simulink library "halout"  (R2021b)
settings: Solver=VariableStepAuto  StartTime=0.0  StopTime=10.0  RelTol=1e-3
undefined symbols (not defined in the file): C_TASK_5MS_S, FALSE, KHAL_CAN1FD1APS3E2E_flg, KHAL_CAN1FD1APS3TxReq_flg, KHAL_CAN1FD1VCU2E2E_flg, KHAL_CAN1FD1VCU2TxReq_flg, KHAL_CAN1FD1VCU3E2E_flg, KHAL_CAN1FD1VCU3TxReq_flg, KHAL_CAN1TxReq_flg, KHAL_CAN1VMCFCM1E2E_flg, KHAL_CAN1VMCFCM1TxReq_flg, KHAL_CAN2TxReq_flg, KHAL_CAN3FD3VCU1toNIDECTxReq_flg, KHAL_CAN3FD3VCU1TxReq_flg, KHAL_CAN3FD3VCU2E2E_flg, KHAL_CAN3FD3VCU2toNIDECE2E_flg, KHAL_CAN3FD3VCU2toNIDECTxReq_flg, KHAL_CAN3FD3VCU2TxReq_flg, KHAL_CAN3TxReq_flg, KHAL_CAN4FD4CE1000E2E_flg, KHAL_CAN4FD4CE1000TxReq_flg, KHAL_CAN4TxReq_flg, KHAL_CAN5TxReq_flg, KHAL_CAN6FD6APS3E2E_flg, KHAL_CAN6FD6APS3TxReq_flg, KHAL_CAN6FD6VCU2E2E_flg, KHAL_CAN6FD6VCU2TxReq_flg, KHAL_CAN6TxReq_flg, ONE_INT, TRUE, ZERO_INT
libraries: FVT_lib x551, simulink x244
(part 15 of 26)

== system halout/HAL_OUT/CAN1/FD1_THCM1_0x182/RrCoolantflow ==
  RrCoolantflow : Inport
  Data Type Conversion : DataTypeConversion  OutDataTypeStr=uint8  RndMeth=Round
  convert_out : FVT_lib/hal/convert_out  gain=0.25  offset=0
  CAN1_Rr_Coolantflow : Outport
  wires:
  Data Type Conversion/1 -> CAN1_Rr_Coolantflow/1
  convert_out/1 -> Data Type Conversion/1
  RrCoolantflow/1 -> convert_out/1

== system halout/HAL_OUT/CAN1/FD1_THCM1_0x182/RrCoolanttemp ==
  RrCoolanttemp : Inport
  Data Type Conversion : DataTypeConversion  OutDataTypeStr=uint16  RndMeth=Round
  convert_out : FVT_lib/hal/convert_out  gain=1  offset=-40
  CAN1_Rr_Coolanttemp : Outport
  wires:
  Data Type Conversion/1 -> CAN1_Rr_Coolanttemp/1
  convert_out/1 -> Data Type Conversion/1
  RrCoolanttemp/1 -> convert_out/1

== system halout/HAL_OUT/CAN1/FD1_THCM1_0x182/sigAirIntenZon1St ==
  sigAirIntenZon1St : Inport
  Data Type Conversion : DataTypeConversion  OutDataTypeStr=uint8  RndMeth=Round
  CAN1_sigAirIntenZon1St : Outport
  wires:
  Data Type Conversion/1 -> CAN1_sigAirIntenZon1St/1
  sigAirIntenZon1St/1 -> Data Type Conversion/1

== system halout/HAL_OUT/CAN1/FD1_THCM1_0x182/sigAirIntenZon3St ==
  sigAirIntenZon3St : Inport
  Data Type Conversion : DataTypeConversion  OutDataTypeStr=uint8  RndMeth=Round
  CAN1_sigAirIntenZon3St : Outport
  wires:
  Data Type Conversion/1 -> CAN1_sigAirIntenZon3St/1
  sigAirIntenZon3St/1 -> Data Type Conversion/1

== system halout/HAL_OUT/CAN1/FD1_THCM1_0x182/sigAmbAirT ==
  sigAmbAirT : Inport
  Data Type Conversion : DataTypeConversion  OutDataTypeStr=uint8  RndMeth=Round
  convert_out : FVT_lib/hal/convert_out  gain=0.5  offset=-40
  CAN1_sigAmbAirT : Outport
  wires:
  Data Type Conversion/1 -> CAN1_sigAmbAirT/1
  convert_out/1 -> Data Type Conversion/1
  sigAmbAirT/1 -> convert_out/1

== system halout/HAL_OUT/CAN1/FD1_THCM1_0x182/sigCbnAirT ==
  sigCbnAirT : Inport
  Data Type Conversion : DataTypeConversion  OutDataTypeStr=uint8  RndMeth=Round
  convert_out : FVT_lib/hal/convert_out  gain=0.5  offset=-40
  CAN1_sigCbnAirT : Outport
  wires:
  Data Type Conversion/1 -> CAN1_sigCbnAirT/1
  convert_out/1 -> Data Type Conversion/1
  sigCbnAirT/1 -> convert_out/1

== system halout/HAL_OUT/CAN1/FD1_THCM1_0x182/sigCbnPTCPwrAct ==
  sigCbnPTCPwrAct : Inport
  Data Type Conversion : DataTypeConversion  OutDataTypeStr=uint8  RndMeth=Round
  convert_out : FVT_lib/hal/convert_out  gain=50  offset=0
  CAN1_sigCbnPTCPwrAct : Outport
  wires:
  Data Type Conversion/1 -> CAN1_sigCbnPTCPwrAct/1
  convert_out/1 -> Data Type Conversion/1
  sigCbnPTCPwrAct/1 -> convert_out/1

== system halout/HAL_OUT/CAN1/FD1_THCM1_0x182/sigCbnSolarLeft ==
  sigCbnSolarLeft : Inport
  Data Type Conversion : DataTypeConversion  OutDataTypeStr=uint8  RndMeth=Round
  convert_out : FVT_lib/hal/convert_out  gain=5  offset=0
  CAN1_sigCbnSolarLeft : Outport
  wires:
  Data Type Conversion/1 -> CAN1_sigCbnSolarLeft/1
  convert_out/1 -> Data Type Conversion/1
  sigCbnSolarLeft/1 -> convert_out/1

== system halout/HAL_OUT/CAN1/FD1_THCM1_0x182/sigCbnSolarRight ==
  sigCbnSolarRight : Inport
  Data Type Conversion : DataTypeConversion  OutDataTypeStr=uint8  RndMeth=Round
  convert_out : FVT_lib/hal/convert_out  gain=5  offset=0
  CAN1_sigCbnSolarRight : Outport
  wires:
  Data Type Conversion/1 -> CAN1_sigCbnSolarRight/1
  convert_out/1 -> Data Type Conversion/1
  sigCbnSolarRight/1 -> convert_out/1

== system halout/HAL_OUT/CAN1/FD1_THCM1_0x182/sigClmtCmprPwrAct ==
  sigClmtCmprPwrAct : Inport
  Data Type Conversion : DataTypeConversion  OutDataTypeStr=uint8  RndMeth=Round
  convert_out : FVT_lib/hal/convert_out  gain=50  offset=0
  CAN1_sigClmtCmprPwrAct : Outport
  wires:
  Data Type Conversion/1 -> CAN1_sigClmtCmprPwrAct/1
  convert_out/1 -> Data Type Conversion/1
  sigClmtCmprPwrAct/1 -> convert_out/1

== system halout/HAL_OUT/CAN1/FD1_THCM1_0x182/sigClntTHvBattOut ==
  sigClntTHvBattOut : Inport
  Data Type Conversion : DataTypeConversion  OutDataTypeStr=uint8  RndMeth=Round
  convert_out : FVT_lib/hal/convert_out  gain=0.5  offset=-40
  CAN1_sigClntTHvBattOut : Outport
  wires:
  Data Type Conversion/1 -> CAN1_sigClntTHvBattOut/1
  convert_out/1 -> Data Type Conversion/1
  sigClntTHvBattOut/1 -> convert_out/1

== system halout/HAL_OUT/CAN1/FD1_THCM1_0x182/sigDfrstSt ==
  sigDfrstSt : Inport
  Data Type Conversion : DataTypeConversion  OutDataTypeStr=uint8  RndMeth=Round
  CAN1_sigDfrstSt : Outport
  wires:
  Data Type Conversion/1 -> CAN1_sigDfrstSt/1
  sigDfrstSt/1 -> Data Type Conversion/1

== system halout/HAL_OUT/CAN1/FD1_THCM1_0x182/sigHvacSt ==
  sigHvacSt : Inport
  Data Type Conversion : DataTypeConversion  OutDataTypeStr=uint8  RndMeth=Round
  CAN1_sigHvacSt : Outport
  wires:
  Data Type Conversion/1 -> CAN1_sigHvacSt/1
  sigHvacSt/1 -> Data Type Conversion/1

== system halout/HAL_OUT/CAN1/FD1_THCM1_0x182/sigRecircSt ==
  sigRecircSt : Inport
  Data Type Conversion : DataTypeConversion  OutDataTypeStr=uint8  RndMeth=Round
  CAN1_sigRecircSt : Outport
  wires:
  Data Type Conversion/1 -> CAN1_sigRecircSt/1
  sigRecircSt/1 -> Data Type Conversion/1

== system halout/HAL_OUT/CAN1/FD1_THCM1_0x182/sigSetTempZon1St ==
  sigSetTempZon1St : Inport
  Data Type Conversion : DataTypeConversion  OutDataTypeStr=uint8  RndMeth=Round
  convert_out : FVT_lib/hal/convert_out  gain=0.5  offset=17
  CAN1_sigSetTempZon1St : Outport
  wires:
  Data Type Conversion/1 -> CAN1_sigSetTempZon1St/1
  convert_out/1 -> Data Type Conversion/1
  sigSetTempZon1St/1 -> convert_out/1

== system halout/HAL_OUT/CAN1/FD1_THCM1_0x182/sigSetTempZon2St ==
  sigSetTempZon2St : Inport
  Data Type Conversion : DataTypeConversion  OutDataTypeStr=uint8  RndMeth=Round
  convert_out : FVT_lib/hal/convert_out  gain=0.5  offset=17
  CAN1_sigSetTempZon2St : Outport
  wires:
  Data Type Conversion/1 -> CAN1_sigSetTempZon2St/1
  convert_out/1 -> Data Type Conversion/1
  sigSetTempZon2St/1 -> convert_out/1

== system halout/HAL_OUT/CAN1/FD1_THCM1_0x182/sigSetTempZon3St ==
  sigSetTempZon3St : Inport
  Data Type Conversion : DataTypeConversion  OutDataTypeStr=uint8  RndMeth=Round
  convert_out : FVT_lib/hal/convert_out  gain=0.5  offset=17
  CAN1_sigSetTempZon3St : Outport
  wires:
  Data Type Conversion/1 -> CAN1_sigSetTempZon3St/1
  convert_out/1 -> Data Type Conversion/1
  sigSetTempZon3St/1 -> convert_out/1

== system halout/HAL_OUT/CAN1/FD1_THCM1_0x182/sigWindDirZon1St ==
  sigWindDirZon1St : Inport
  Data Type Conversion : DataTypeConversion  OutDataTypeStr=uint8  RndMeth=Round
  CAN1_sigWindDirZon1St : Outport
  wires:
  Data Type Conversion/1 -> CAN1_sigWindDirZon1St/1
  sigWindDirZon1St/1 -> Data Type Conversion/1

== system halout/HAL_OUT/CAN1/FD1_THCM1_0x182/sigWindDirZon3St ==
  sigWindDirZon3St : Inport
  Data Type Conversion : DataTypeConversion  OutDataTypeStr=uint8  RndMeth=Round
  CAN1_sigWindDirZon3St : Outport
  wires:
  Data Type Conversion/1 -> CAN1_sigWindDirZon3St/1
  sigWindDirZon3St/1 -> Data Type Conversion/1

== system halout/HAL_OUT/CAN1/FD1_VCU1_0x116/CCCrlSta ==
  CCCrlSta : Inport
  Data Type Conversion : DataTypeConversion  OutDataTypeStr=uint8  RndMeth=Round
  CAN1_CC_Crl_Sta : Outport
  wires:
  Data Type Conversion/1 -> CAN1_CC_Crl_Sta/1
  CCCrlSta/1 -> Data Type Conversion/1

== system halout/HAL_OUT/CAN1/FD1_VCU1_0x116/EngAGSCloseSta ==
  EngAGSCloseSta : Inport
  Data Type Conversion : DataTypeConversion  OutDataTypeStr=uint8  RndMeth=Round
  CAN1_Eng_AGSCloseSta : Outport
  wires:
  Data Type Conversion/1 -> CAN1_Eng_AGSCloseSta/1
  EngAGSCloseSta/1 -> Data Type Conversion/1

== system halout/HAL_OUT/CAN1/FD1_VCU1_0x116/EngActvDmpDisabSta ==
  EngActvDmpDisabSta : Inport
  Data Type Conversion : DataTypeConversion  OutDataTypeStr=uint8  RndMeth=Round
  CAN1_Eng_ActvDmpDisabSta : Outport
  wires:
  Data Type Conversion/1 -> CAN1_Eng_ActvDmpDisabSta/1
  EngActvDmpDisabSta/1 -> Data Type Conversion/1

== system halout/HAL_OUT/CAN1/FD1_VCU1_0x116/EngCoastDwSta ==
  EngCoastDwSta : Inport
  Data Type Conversion : DataTypeConversion  OutDataTypeStr=uint8  RndMeth=Round
  CAN1_Eng_CoastDwSta : Outport
  wires:
  Data Type Conversion/1 -> CAN1_Eng_CoastDwSta/1
  EngCoastDwSta/1 -> Data Type Conversion/1

== system halout/HAL_OUT/CAN1/FD1_VCU1_0x116/EngPwrLockSta ==
  EngPwrLockSta : Inport
  Data Type Conversion : DataTypeConversion  OutDataTypeStr=uint8  RndMeth=Round
  CAN1_Eng_PwrLockSta : Outport
  wires:
  Data Type Conversion/1 -> CAN1_Eng_PwrLockSta/1
  EngPwrLockSta/1 -> Data Type Conversion/1

== system halout/HAL_OUT/CAN1/FD1_VCU1_0x116/HVPwrSta ==
  HVPwrSta : Inport
  Data Type Conversion : DataTypeConversion  OutDataTypeStr=uint8  RndMeth=Round
  CAN1_HVPwrSta : Outport
  wires:
  Data Type Conversion/1 -> CAN1_HVPwrSta/1
  HVPwrSta/1 -> Data Type Conversion/1

== system halout/HAL_OUT/CAN1/FD1_VCU1_0x116/LVPwrSta ==
  LVPwrSta : Inport
  Data Type Conversion : DataTypeConversion  OutDataTypeStr=uint8  RndMeth=Round
  CAN1_LVPwrSta : Outport
  wires:
  Data Type Conversion/1 -> CAN1_LVPwrSta/1
  LVPwrSta/1 -> Data Type Conversion/1

== system halout/HAL_OUT/CAN1/FD1_VCU1_0x116/MSACrlSta ==
  MSACrlSta : Inport
  Data Type Conversion : DataTypeConversion  OutDataTypeStr=uint8  RndMeth=Round
  CAN1_MSA_Crl_Sta : Outport
  wires:
  Data Type Conversion/1 -> CAN1_MSA_Crl_Sta/1
  MSACrlSta/1 -> Data Type Conversion/1

== system halout/HAL_OUT/CAN1/FD1_VCU1_0x116/PButtonSta ==
  PButtonSta : Inport
  Data Type Conversion : DataTypeConversion  OutDataTypeStr=uint8  RndMeth=Round
  CAN1_P_Button_Sta : Outport
  wires:
  Data Type Conversion/1 -> CAN1_P_Button_Sta/1
  PButtonSta/1 -> Data Type Conversion/1

== system halout/HAL_OUT/CAN1/FD1_VCU1_0x116/PrkReq ==
  PrkReq : Inport
  Data Type Conversion : DataTypeConversion  OutDataTypeStr=uint8  RndMeth=Round
  CAN1_PrkReq : Outport
  wires:
  Data Type Conversion/1 -> CAN1_PrkReq/1
  PrkReq/1 -> Data Type Conversion/1

== system halout/HAL_OUT/CAN1/FD1_VCU1_0x116/PrkReqValid ==
  PrkReqValid : Inport
  Data Type Conversion : DataTypeConversion  OutDataTypeStr=uint8  RndMeth=Round
  CAN1_PrkReqValid : Outport
  wires:
  Data Type Conversion/1 -> CAN1_PrkReqValid/1
  PrkReqValid/1 -> Data Type Conversion/1

== system halout/HAL_OUT/CAN1/FD1_VCU1_0x116/PwrSta ==
  PwrSta : Inport
  Data Type Conversion : DataTypeConversion  OutDataTypeStr=uint8  RndMeth=Round
  CAN1_PwrSta : Outport
  wires:
  Data Type Conversion/1 -> CAN1_PwrSta/1
  PwrSta/1 -> Data Type Conversion/1

== system halout/HAL_OUT/CAN1/FD1_VCU1_0x116/ShiftGearPosn ==
  ShiftGearPosn : Inport
  Data Type Conversion : DataTypeConversion  OutDataTypeStr=uint8  RndMeth=Round
  CAN1_ShiftGearPosn : Outport
  wires:
  Data Type Conversion/1 -> CAN1_ShiftGearPosn/1
  ShiftGearPosn/1 -> Data Type Conversion/1

== system halout/HAL_OUT/CAN1/FD1_VCU1_0x116/VehMalfunLevel ==
  VehMalfunLevel : Inport
  Data Type Conversion : DataTypeConversion  OutDataTypeStr=uint8  RndMeth=Round
  CAN1_VehMalfunLevel : Outport
  wires:
  Data Type Conversion/1 -> CAN1_VehMalfunLevel/1
  VehMalfunLevel/1 -> Data Type Conversion/1

== system halout/HAL_OUT/CAN1/FD1_VCU1_0x116/XWDMode ==
  XWDMode : Inport
  Data Type Conversion : DataTypeConversion  OutDataTypeStr=uint8  RndMeth=Round
  CAN1_XWDMode : Outport
  wires:
  Data Type Conversion/1 -> CAN1_XWDMode/1
  XWDMode/1 -> Data Type Conversion/1

== system halout/HAL_OUT/CAN1/FD1_VCU2_0x154/ACCCtrlAvail ==
  ACCCtrlAvail : Inport
  Data Type Conversion : DataTypeConversion  OutDataTypeStr=uint8  RndMeth=Round
  CAN1_ACC_CtrlAvail : Outport
  wires:
  Data Type Conversion/1 -> CAN1_ACC_CtrlAvail/1
  ACCCtrlAvail/1 -> Data Type Conversion/1

== system halout/HAL_OUT/CAN1/FD1_VCU2_0x154/AccPedalOverride ==
  AccPedalOverride : Inport
  Data Type Conversion : DataTypeConversion  OutDataTypeStr=uint8  RndMeth=Round
  CAN1_AccPedal_Override : Outport
  wires:
  Data Type Conversion/1 -> CAN1_AccPedal_Override/1
  AccPedalOverride/1 -> Data Type Conversion/1

== system halout/HAL_OUT/CAN1/FD1_VCU2_0x154/ActAPSPosn ==
  ActAPSPosn : Inport
  Data Type Conversion : DataTypeConversion  OutDataTypeStr=uint8  RndMeth=Round
  convert_out : FVT_lib/hal/convert_out  gain=0.394  offset=0
  CAN1_ActAPSPosn : Outport
  wires:
  Data Type Conversion/1 -> CAN1_ActAPSPosn/1
  convert_out/1 -> Data Type Conversion/1
  ActAPSPosn/1 -> convert_out/1

== system halout/HAL_OUT/CAN1/FD1_VCU2_0x154/Byte_0 ==
  CS_VCU2_CAN1 : Inport
  BitwiseOR : simulink/Logic and Bit Operations/Bitwise Operator  logicop=OR  UseBitMask=off  BitMask=bin2dec('11011001')  BitMaskRealWorld=Stored Integer
  SignalPack : FVT_lib/hal/SignalPack  RightShiftCnt=0  BitMask=2^8-1  LeftShiftCnt=0
  UnitConverter : DataTypeConversion  OutDataTypeStr=uint8  RndMeth=Round
  UnitConverter1 : DataTypeConversion  OutDataTypeStr=uint8  RndMeth=Round
  Byte_0 : Outport
  wires:
  BitwiseOR/1 -> Byte_0/1
  UnitConverter/1 -> BitwiseOR/1
  SignalPack/1 -> UnitConverter/1
  UnitConverter1/1 -> SignalPack/1
  CS_VCU2_CAN1/1 -> UnitConverter1/1

== system halout/HAL_OUT/CAN1/FD1_VCU2_0x154/Byte_1 ==
  RC_VCU2_CAN1 : Inport
  BitwiseOR : simulink/Logic and Bit Operations/Bitwise Operator  logicop=OR  UseBitMask=off  BitMask=bin2dec('11011001')  BitMaskRealWorld=Stored Integer
  SignalPack : FVT_lib/hal/SignalPack  RightShiftCnt=0  BitMask=2^4-1  LeftShiftCnt=0
  UnitConverter : DataTypeConversion  OutDataTypeStr=uint8  RndMeth=Round
  UnitConverter1 : DataTypeConversion  OutDataTypeStr=uint8  RndMeth=Round
  Byte_1 : Outport
  wires:
  BitwiseOR/1 -> Byte_1/1
  UnitConverter/1 -> BitwiseOR/1
  SignalPack/1 -> UnitConverter/1
  UnitConverter1/1 -> SignalPack/1
  RC_VCU2_CAN1/1 -> UnitConverter1/1

== system halout/HAL_OUT/CAN1/FD1_VCU2_0x154/Byte_10 ==
  VehActPwr : Inport
  BitwiseOR : simulink/Logic and Bit Operations/Bitwise Operator  logicop=OR  UseBitMask=off  BitMask=bin2dec('11011001')  BitMaskRealWorld=Stored Integer
  SignalPack : FVT_lib/hal/SignalPack  RightShiftCnt=16  BitMask=2^8-1  LeftShiftCnt=0
  UnitConverter : DataTypeConversion  OutDataTypeStr=uint8  RndMeth=Round
  UnitConverter1 : DataTypeConversion  OutDataTypeStr=uint32  RndMeth=Round
  convert_out : FVT_lib/hal/convert_out  gain=1  offset=-600000
  Byte_10 : Outport
  wires:
  BitwiseOR/1 -> Byte_10/1
  UnitConverter/1 -> BitwiseOR/1
  SignalPack/1 -> UnitConverter/1
  UnitConverter1/1 -> SignalPack/1
  convert_out/1 -> UnitConverter1/1
  VehActPwr/1 -> convert_out/1

== system halout/HAL_OUT/CAN1/FD1_VCU2_0x154/Byte_11 ==
  VehActPwr : Inport
  BitwiseOR : simulink/Logic and Bit Operations/Bitwise Operator  logicop=OR  UseBitMask=off  BitMask=bin2dec('11011001')  BitMaskRealWorld=Stored Integer
  SignalPack : FVT_lib/hal/SignalPack  RightShiftCnt=8  BitMask=2^8-1  LeftShiftCnt=0
  UnitConverter : DataTypeConversion  OutDataTypeStr=uint8  RndMeth=Round
  UnitConverter1 : DataTypeConversion  OutDataTypeStr=uint32  RndMeth=Round
  convert_out : FVT_lib/hal/convert_out  gain=1  offset=-600000
  Byte_11 : Outport
  wires:
  BitwiseOR/1 -> Byte_11/1
  UnitConverter/1 -> BitwiseOR/1
  SignalPack/1 -> UnitConverter/1
  UnitConverter1/1 -> SignalPack/1
  convert_out/1 -> UnitConverter1/1
  VehActPwr/1 -> convert_out/1

== system halout/HAL_OUT/CAN1/FD1_VCU2_0x154/Byte_12 ==
  VehActPwr : Inport
  BitwiseOR : simulink/Logic and Bit Operations/Bitwise Operator  logicop=OR  UseBitMask=off  BitMask=bin2dec('11011001')  BitMaskRealWorld=Stored Integer
  SignalPack : FVT_lib/hal/SignalPack  RightShiftCnt=0  BitMask=2^8-1  LeftShiftCnt=0
  UnitConverter : DataTypeConversion  OutDataTypeStr=uint8  RndMeth=Round
  UnitConverter1 : DataTypeConversion  OutDataTypeStr=uint32  RndMeth=Round
  convert_out : FVT_lib/hal/convert_out  gain=1  offset=-600000
  Byte_12 : Outport
  wires:
  BitwiseOR/1 -> Byte_12/1
  UnitConverter/1 -> BitwiseOR/1
  SignalPack/1 -> UnitConverter/1
  UnitConverter1/1 -> SignalPack/1
  convert_out/1 -> UnitConverter1/1
  VehActPwr/1 -> convert_out/1

== system halout/HAL_OUT/CAN1/FD1_VCU2_0x154/Byte_13 ==
  DriverTq : Inport
  BitwiseOR : simulink/Logic and Bit Operations/Bitwise Operator  logicop=OR  UseBitMask=off  BitMask=bin2dec('11011001')  BitMaskRealWorld=Stored Integer
  SignalPack : FVT_lib/hal/SignalPack  RightShiftCnt=8  BitMask=2^8-1  LeftShiftCnt=0
  UnitConverter : DataTypeConversion  OutDataTypeStr=uint8  RndMeth=Round
  UnitConverter1 : DataTypeConversion  OutDataTypeStr=uint16  RndMeth=Round
  convert_out : FVT_lib/hal/convert_out  gain=1  offset=-4300
  Byte_13 : Outport
  wires:
  BitwiseOR/1 -> Byte_13/1
  UnitConverter/1 -> BitwiseOR/1
  SignalPack/1 -> UnitConverter/1
  UnitConverter1/1 -> SignalPack/1
  convert_out/1 -> UnitConverter1/1
  DriverTq/1 -> convert_out/1

== system halout/HAL_OUT/CAN1/FD1_VCU2_0x154/Byte_14 ==
  DriverTq : Inport
  BitwiseOR : simulink/Logic and Bit Operations/Bitwise Operator  logicop=OR  UseBitMask=off  BitMask=bin2dec('11011001')  BitMaskRealWorld=Stored Integer
  SignalPack : FVT_lib/hal/SignalPack  RightShiftCnt=0  BitMask=2^8-1  LeftShiftCnt=0
  UnitConverter : DataTypeConversion  OutDataTypeStr=uint8  RndMeth=Round
  UnitConverter1 : DataTypeConversion  OutDataTypeStr=uint16  RndMeth=Round
  convert_out : FVT_lib/hal/convert_out  gain=1  offset=-4300
  Byte_14 : Outport
  wires:
  BitwiseOR/1 -> Byte_14/1
  UnitConverter/1 -> BitwiseOR/1
  SignalPack/1 -> UnitConverter/1
  UnitConverter1/1 -> SignalPack/1
  convert_out/1 -> UnitConverter1/1
  DriverTq/1 -> convert_out/1

== system halout/HAL_OUT/CAN1/FD1_VCU2_0x154/Byte_15 ==
  ActAPSPosn : Inport
  BitwiseOR : simulink/Logic and Bit Operations/Bitwise Operator  logicop=OR  UseBitMask=off  BitMask=bin2dec('11011001')  BitMaskRealWorld=Stored Integer
  SignalPack : FVT_lib/hal/SignalPack  RightShiftCnt=0  BitMask=2^8-1  LeftShiftCnt=0
  UnitConverter : DataTypeConversion  OutDataTypeStr=uint8  RndMeth=Round
  UnitConverter1 : DataTypeConversion  OutDataTypeStr=uint8  RndMeth=Round
  convert_out : FVT_lib/hal/convert_out  gain=0.394  offset=0
  Byte_15 : Outport
  wires:
  BitwiseOR/1 -> Byte_15/1
  UnitConverter/1 -> BitwiseOR/1
  SignalPack/1 -> UnitConverter/1
  UnitConverter1/1 -> SignalPack/1
  convert_out/1 -> UnitConverter1/1
  ActAPSPosn/1 -> convert_out/1

== system halout/HAL_OUT/CAN1/FD1_VCU2_0x154/Byte_2 ==
  Fr_DriverTq : Inport
  BitwiseOR : simulink/Logic and Bit Operations/Bitwise Operator  logicop=OR  UseBitMask=off  BitMask=bin2dec('11011001')  BitMaskRealWorld=Stored Integer
  SignalPack : FVT_lib/hal/SignalPack  RightShiftCnt=8  BitMask=2^8-1  LeftShiftCnt=0
  UnitConverter : DataTypeConversion  OutDataTypeStr=uint8  RndMeth=Round
  UnitConverter1 : DataTypeConversion  OutDataTypeStr=uint16  RndMeth=Round
  convert_out : FVT_lib/hal/convert_out  gain=0.5  offset=-5300
  Byte_2 : Outport
  wires:
  BitwiseOR/1 -> Byte_2/1
  UnitConverter/1 -> BitwiseOR/1
  SignalPack/1 -> UnitConverter/1
  UnitConverter1/1 -> SignalPack/1
  convert_out/1 -> UnitConverter1/1
  Fr_DriverTq/1 -> convert_out/1

== system halout/HAL_OUT/CAN1/FD1_VCU2_0x154/Byte_3 ==
  Fr_DriverTq : Inport
  BitwiseOR : simulink/Logic and Bit Operations/Bitwise Operator  logicop=OR  UseBitMask=off  BitMask=bin2dec('11011001')  BitMaskRealWorld=Stored Integer
  SignalPack : FVT_lib/hal/SignalPack  RightShiftCnt=0  BitMask=2^8-1  LeftShiftCnt=0
  UnitConverter : DataTypeConversion  OutDataTypeStr=uint8  RndMeth=Round
  UnitConverter1 : DataTypeConversion  OutDataTypeStr=uint16  RndMeth=Round
  convert_out : FVT_lib/hal/convert_out  gain=0.5  offset=-5300
  Byte_3 : Outport
  wires:
  BitwiseOR/1 -> Byte_3/1
  UnitConverter/1 -> BitwiseOR/1
  SignalPack/1 -> UnitConverter/1
  UnitConverter1/1 -> SignalPack/1
  convert_out/1 -> UnitConverter1/1
  Fr_DriverTq/1 -> convert_out/1

== system halout/HAL_OUT/CAN1/FD1_VCU2_0x154/Byte_4 ==
  Rr_DriverTq : Inport
  BitwiseOR : simulink/Logic and Bit Operations/Bitwise Operator  logicop=OR  UseBitMask=off  BitMask=bin2dec('11011001')  BitMaskRealWorld=Stored Integer
  SignalPack : FVT_lib/hal/SignalPack  RightShiftCnt=8  BitMask=2^8-1  LeftShiftCnt=0
  UnitConverter : DataTypeConversion  OutDataTypeStr=uint8  RndMeth=Round
  UnitConverter1 : DataTypeConversion  OutDataTypeStr=uint16  RndMeth=Round
  convert_out : FVT_lib/hal/convert_out  gain=0.5  offset=-5300
  Byte_4 : Outport
  wires:
  BitwiseOR/1 -> Byte_4/1
  UnitConverter/1 -> BitwiseOR/1
  SignalPack/1 -> UnitConverter/1
  UnitConverter1/1 -> SignalPack/1
  convert_out/1 -> UnitConverter1/1
  Rr_DriverTq/1 -> convert_out/1

== system halout/HAL_OUT/CAN1/FD1_VCU2_0x154/Byte_5 ==
  Rr_DriverTq : Inport
  BitwiseOR : simulink/Logic and Bit Operations/Bitwise Operator  logicop=OR  UseBitMask=off  BitMask=bin2dec('11011001')  BitMaskRealWorld=Stored Integer
  SignalPack : FVT_lib/hal/SignalPack  RightShiftCnt=0  BitMask=2^8-1  LeftShiftCnt=0
  UnitConverter : DataTypeConversion  OutDataTypeStr=uint8  RndMeth=Round
  UnitConverter1 : DataTypeConversion  OutDataTypeStr=uint16  RndMeth=Round
  convert_out : FVT_lib/hal/convert_out  gain=0.5  offset=-5300
  Byte_5 : Outport
  wires:
  BitwiseOR/1 -> Byte_5/1
  UnitConverter/1 -> BitwiseOR/1
  SignalPack/1 -> UnitConverter/1
  UnitConverter1/1 -> SignalPack/1
  convert_out/1 -> UnitConverter1/1
  Rr_DriverTq/1 -> convert_out/1

== system halout/HAL_OUT/CAN1/FD1_VCU2_0x154/Byte_6 ==
  ACC_CtrlAvail : Inport
  AccPedal_Override : Inport  Port=2
  BitwiseOR : simulink/Logic and Bit Operations/Bitwise Operator  logicop=OR  UseBitMask=off  NumInputPorts=2  BitMask=bin2dec('11011001')  BitMaskRealWorld=Stored Integer
  SignalPack : FVT_lib/hal/SignalPack  RightShiftCnt=0  BitMask=2^1-1  LeftShiftCnt=7
  SignalPack1 : FVT_lib/hal/SignalPack  RightShiftCnt=0  BitMask=2^1-1  LeftShiftCnt=6
  UnitConverter{,1..3} (4 alike) : DataTypeConversion  OutDataTypeStr=uint8  RndMeth=Round
  Byte_6 : Outport
  wires:
  BitwiseOR/1 -> Byte_6/1
  UnitConverter/1 -> BitwiseOR/1
  SignalPack/1 -> UnitConverter/1
  UnitConverter1/1 -> SignalPack/1
  ACC_CtrlAvail/1 -> UnitConverter1/1
  UnitConverter2/1 -> BitwiseOR/2
  SignalPack1/1 -> UnitConverter2/1
  UnitConverter3/1 -> SignalPack1/1
  AccPedal_Override/1 -> UnitConverter3/1

== system halout/HAL_OUT/CAN1/FD1_VCU2_0x154/CRC8_IfAction_Tx ==
  CAN_E2E_flg : Inport
  DataID1 : Inport  Port=2
  DataID2 : Inport  Port=3
  RawData : Inport  Port=4
  Data Type Conversion : DataTypeConversion  OutDataTypeStr=uint8
  If : If
  If Action Subsystem : Subsystem  TreatAsAtomicUnit=on
  If Action Subsystem1 : Subsystem  TreatAsAtomicUnit=on
  Merge : Merge
  CRC8 : Outport
  wires:
  If/2 -> If Action Subsystem/Action
  If/1 -> If Action Subsystem1/Action
  CAN_E2E_flg/1 -> [CAN_E2E_flg]
  DataID1/1 -> [DataID1]
  DataID2/1 -> [DataID2]
  RawData/1 -> [RawData]
  [CAN_E2E_flg] -> Data Type Conversion/1
  [DataID1] -> If Action Subsystem1/1(CAN_E2E_ID1)
  [DataID2] -> If Action Subsystem1/2(CAN_E2E_ID2)
  [RawData] -> If Action Subsystem1/3(Byte1)
  [RawData] -> If Action Subsystem/1(Byte1)
  If Action Subsystem1/1(CRC8_E2EResult) -> Merge/1
  If Action Subsystem/1(CRC8_Result) -> Merge/2
  Merge/1 -> CRC8/1
  Data Type Conversion/1 -> If/1

== system halout/HAL_OUT/CAN1/FD1_VCU2_0x154/CSVCU2CAN1 ==
  CSVCU2CAN1 : Inport
  Data Type Conversion : DataTypeConversion  OutDataTypeStr=uint8  RndMeth=Round
  CAN1_CS_VCU2_CAN1 : Outport
  wires:
  Data Type Conversion/1 -> CAN1_CS_VCU2_CAN1/1
  CSVCU2CAN1/1 -> Data Type Conversion/1

== system halout/HAL_OUT/CAN1/FD1_VCU2_0x154/DriverTq ==
  DriverTq : Inport
  Data Type Conversion : DataTypeConversion  OutDataTypeStr=uint16  RndMeth=Round
  convert_out : FVT_lib/hal/convert_out  gain=1  offset=-4300
  CAN1_DriverTq : Outport
  wires:
  Data Type Conversion/1 -> CAN1_DriverTq/1
  convert_out/1 -> Data Type Conversion/1
  DriverTq/1 -> convert_out/1

== system halout/HAL_OUT/CAN1/FD1_VCU2_0x154/FrDriverTq ==
  FrDriverTq : Inport
  Data Type Conversion : DataTypeConversion  OutDataTypeStr=uint16  RndMeth=Round
  convert_out : FVT_lib/hal/convert_out  gain=0.5  offset=-5300
  CAN1_Fr_DriverTq : Outport
  wires:
  Data Type Conversion/1 -> CAN1_Fr_DriverTq/1
  convert_out/1 -> Data Type Conversion/1
  FrDriverTq/1 -> convert_out/1

== system halout/HAL_OUT/CAN1/FD1_VCU2_0x154/RCVCU2CAN1 ==
  RCVCU2CAN1 : Inport
  Data Type Conversion : DataTypeConversion  OutDataTypeStr=uint8  RndMeth=Round
  CAN1_RC_VCU2_CAN1 : Outport
  wires:
  Data Type Conversion/1 -> CAN1_RC_VCU2_CAN1/1
  RCVCU2CAN1/1 -> Data Type Conversion/1

== system halout/HAL_OUT/CAN1/FD1_VCU2_0x154/RrDriverTq ==
  RrDriverTq : Inport
  Data Type Conversion : DataTypeConversion  OutDataTypeStr=uint16  RndMeth=Round
  convert_out : FVT_lib/hal/convert_out  gain=0.5  offset=-5300
  CAN1_Rr_DriverTq : Outport
  wires:
  Data Type Conversion/1 -> CAN1_Rr_DriverTq/1
  convert_out/1 -> Data Type Conversion/1
  RrDriverTq/1 -> convert_out/1

== system halout/HAL_OUT/CAN1/FD1_VCU2_0x154/VehActPwr ==
  VehActPwr : Inport
  Data Type Conversion : DataTypeConversion  OutDataTypeStr=uint32  RndMeth=Round
  convert_out : FVT_lib/hal/convert_out  gain=1  offset=-600000
  CAN1_VehActPwr : Outport
  wires:
  Data Type Conversion/1 -> CAN1_VehActPwr/1
  convert_out/1 -> Data Type Conversion/1
  VehActPwr/1 -> convert_out/1

== system halout/HAL_OUT/CAN1/FD1_VCU3_0x159/Byte_0 ==
  CS_VCU3_CAN1 : Inport
  BitwiseOR : simulink/Logic and Bit Operations/Bitwise Operator  logicop=OR  UseBitMask=off  BitMask=bin2dec('11011001')  BitMaskRealWorld=Stored Integer
  SignalPack : FVT_lib/hal/SignalPack  RightShiftCnt=0  BitMask=2^8-1  LeftShiftCnt=0
  UnitConverter : DataTypeConversion  OutDataTypeStr=uint8  RndMeth=Round
  UnitConverter1 : DataTypeConversion  OutDataTypeStr=uint8  RndMeth=Round
  Byte_0 : Outport
  wires:
  BitwiseOR/1 -> Byte_0/1
  UnitConverter/1 -> BitwiseOR/1
  SignalPack/1 -> UnitConverter/1
  UnitConverter1/1 -> SignalPack/1
  CS_VCU3_CAN1/1 -> UnitConverter1/1

== system halout/HAL_OUT/CAN1/FD1_VCU3_0x159/Byte_1 ==
  RC_VCU3_CAN1 : Inport
  BitwiseOR : simulink/Logic and Bit Operations/Bitwise Operator  logicop=OR  UseBitMask=off  BitMask=bin2dec('11011001')  BitMaskRealWorld=Stored Integer
  SignalPack : FVT_lib/hal/SignalPack  RightShiftCnt=0  BitMask=2^4-1  LeftShiftCnt=0
  UnitConverter : DataTypeConversion  OutDataTypeStr=uint8  RndMeth=Round
  UnitConverter1 : DataTypeConversion  OutDataTypeStr=uint8  RndMeth=Round
  Byte_1 : Outport
  wires:
  BitwiseOR/1 -> Byte_1/1
  UnitConverter/1 -> BitwiseOR/1
  SignalPack/1 -> UnitConverter/1
  UnitConverter1/1 -> SignalPack/1
  RC_VCU3_CAN1/1 -> UnitConverter1/1

== system halout/HAL_OUT/CAN1/FD1_VCU3_0x159/Byte_10 ==
  Rr_EDURealDrvOrBRgnTq : Inport
  BitwiseOR : simulink/Logic and Bit Operations/Bitwise Operator  logicop=OR  UseBitMask=off  BitMask=bin2dec('11011001')  BitMaskRealWorld=Stored Integer
  SignalPack : FVT_lib/hal/SignalPack  RightShiftCnt=8  BitMask=2^8-1  LeftShiftCnt=0
  UnitConverter : DataTypeConversion  OutDataTypeStr=uint8  RndMeth=Round
  UnitConverter1 : DataTypeConversion  OutDataTypeStr=uint16  RndMeth=Round
  convert_out : FVT_lib/hal/convert_out  gain=0.5  offset=-5300
  Byte_10 : Outport
  wires:
  BitwiseOR/1 -> Byte_10/1
  UnitConverter/1 -> BitwiseOR/1
  SignalPack/1 -> UnitConverter/1
  UnitConverter1/1 -> SignalPack/1
  convert_out/1 -> UnitConverter1/1
  Rr_EDURealDrvOrBRgnTq/1 -> convert_out/1

== system halout/HAL_OUT/CAN1/FD1_VCU3_0x159/Byte_11 ==
  Rr_EDURealDrvOrBRgnTq : Inport
  BitwiseOR : simulink/Logic and Bit Operations/Bitwise Operator  logicop=OR  UseBitMask=off  BitMask=bin2dec('11011001')  BitMaskRealWorld=Stored Integer
  SignalPack : FVT_lib/hal/SignalPack  RightShiftCnt=0  BitMask=2^8-1  LeftShiftCnt=0
  UnitConverter : DataTypeConversion  OutDataTypeStr=uint8  RndMeth=Round
  UnitConverter1 : DataTypeConversion  OutDataTypeStr=uint16  RndMeth=Round
  convert_out : FVT_lib/hal/convert_out  gain=0.5  offset=-5300
  Byte_11 : Outport
  wires:
  BitwiseOR/1 -> Byte_11/1
  UnitConverter/1 -> BitwiseOR/1
  SignalPack/1 -> UnitConverter/1
  UnitConverter1/1 -> SignalPack/1
  convert_out/1 -> UnitConverter1/1
  Rr_EDURealDrvOrBRgnTq/1 -> convert_out/1

== system halout/HAL_OUT/CAN1/FD1_VCU3_0x159/Byte_12 ==
  Fr_EDUAvailBrkRgnTqValid : Inport
  Fr_EDUSpd : Inport  Port=2
  Rr_EDUAvailBrkRgnTqValid : Inport  Port=3
  BitwiseOR : simulink/Logic and Bit Operations/Bitwise Operator  logicop=OR  UseBitMask=off  NumInputPorts=3  BitMask=bin2dec('11011001')  BitMaskRealWorld=Stored Integer
  SignalPack : FVT_lib/hal/SignalPack  RightShiftCnt=0  BitMask=2^1-1  LeftShiftCnt=6
  SignalPack1 : FVT_lib/hal/SignalPack  RightShiftCnt=8  BitMask=2^4-1  LeftShiftCnt=0
  SignalPack2 : FVT_lib/hal/SignalPack  RightShiftCnt=0  BitMask=2^1-1  LeftShiftCnt=7
  UnitConverter{,1..2,4..5} (5 alike) : DataTypeConversion  OutDataTypeStr=uint8  RndMeth=Round
  UnitConverter3 : DataTypeConversion  OutDataTypeStr=uint16  RndMeth=Round
  convert_out : FVT_lib/hal/convert_out  gain=1  offset=-2000
  Byte_12 : Outport
  wires:
  BitwiseOR/1 -> Byte_12/1
  UnitConverter/1 -> BitwiseOR/1
  SignalPack/1 -> UnitConverter/1
  UnitConverter1/1 -> SignalPack/1
  Fr_EDUAvailBrkRgnTqValid/1 -> UnitConverter1/1
  UnitConverter2/1 -> BitwiseOR/2
  SignalPack1/1 -> UnitConverter2/1
  UnitConverter3/1 -> SignalPack1/1
  convert_out/1 -> UnitConverter3/1
  Fr_EDUSpd/1 -> convert_out/1
  UnitConverter4/1 -> BitwiseOR/3
  SignalPack2/1 -> UnitConverter4/1
  UnitConverter5/1 -> SignalPack2/1
  Rr_EDUAvailBrkRgnTqValid/1 -> UnitConverter5/1

== system halout/HAL_OUT/CAN1/FD1_VCU3_0x159/Byte_13 ==
  Fr_EDUSpd : Inport
  BitwiseOR : simulink/Logic and Bit Operations/Bitwise Operator  logicop=OR  UseBitMask=off  BitMask=bin2dec('11011001')  BitMaskRealWorld=Stored Integer
  SignalPack : FVT_lib/hal/SignalPack  RightShiftCnt=0  BitMask=2^8-1  LeftShiftCnt=0
  UnitConverter : DataTypeConversion  OutDataTypeStr=uint8  RndMeth=Round
  UnitConverter1 : DataTypeConversion  OutDataTypeStr=uint16  RndMeth=Round
  convert_out : FVT_lib/hal/convert_out  gain=1  offset=-2000
  Byte_13 : Outport
  wires:
  BitwiseOR/1 -> Byte_13/1
  UnitConverter/1 -> BitwiseOR/1
  SignalPack/1 -> UnitConverter/1
  UnitConverter1/1 -> SignalPack/1
  convert_out/1 -> UnitConverter1/1
  Fr_EDUSpd/1 -> convert_out/1

== system halout/HAL_OUT/CAN1/FD1_VCU3_0x159/Byte_14 ==
  Fr_EDURealARgnTq : Inport
  BitwiseOR : simulink/Logic and Bit Operations/Bitwise Operator  logicop=OR  UseBitMask=off  BitMask=bin2dec('11011001')  BitMaskRealWorld=Stored Integer
  SignalPack : FVT_lib/hal/SignalPack  RightShiftCnt=8  BitMask=2^8-1  LeftShiftCnt=0
  UnitConverter : DataTypeConversion  OutDataTypeStr=uint8  RndMeth=Round
  UnitConverter1 : DataTypeConversion  OutDataTypeStr=uint16  RndMeth=Round
  convert_out : FVT_lib/hal/convert_out  gain=1  offset=-5300
  Byte_14 : Outport
  wires:
  BitwiseOR/1 -> Byte_14/1
  UnitConverter/1 -> BitwiseOR/1
  SignalPack/1 -> UnitConverter/1
  UnitConverter1/1 -> SignalPack/1
  convert_out/1 -> UnitConverter1/1
  Fr_EDURealARgnTq/1 -> convert_out/1

== system halout/HAL_OUT/CAN1/FD1_VCU3_0x159/Byte_15 ==
  Fr_EDURealARgnTq : Inport
  BitwiseOR : simulink/Logic and Bit Operations/Bitwise Operator  logicop=OR  UseBitMask=off  BitMask=bin2dec('11011001')  BitMaskRealWorld=Stored Integer
  SignalPack : FVT_lib/hal/SignalPack  RightShiftCnt=0  BitMask=2^8-1  LeftShiftCnt=0
  UnitConverter : DataTypeConversion  OutDataTypeStr=uint8  RndMeth=Round
  UnitConverter1 : DataTypeConversion  OutDataTypeStr=uint16  RndMeth=Round
  convert_out : FVT_lib/hal/convert_out  gain=1  offset=-5300
  Byte_15 : Outport
  wires:
  BitwiseOR/1 -> Byte_15/1
  UnitConverter/1 -> BitwiseOR/1
  SignalPack/1 -> UnitConverter/1
  UnitConverter1/1 -> SignalPack/1
  convert_out/1 -> UnitConverter1/1
  Fr_EDURealARgnTq/1 -> convert_out/1

== system halout/HAL_OUT/CAN1/FD1_VCU3_0x159/Byte_16 ==
  Fr_EDUAvailBrkRgnTq : Inport
  BitwiseOR : simulink/Logic and Bit Operations/Bitwise Operator  logicop=OR  UseBitMask=off  BitMask=bin2dec('11011001')  BitMaskRealWorld=Stored Integer
  SignalPack : FVT_lib/hal/SignalPack  RightShiftCnt=8  BitMask=2^8-1  LeftShiftCnt=0
  UnitConverter : DataTypeConversion  OutDataTypeStr=uint8  RndMeth=Round
  UnitConverter1 : DataTypeConversion  OutDataTypeStr=uint16  RndMeth=Round
  convert_out : FVT_lib/hal/convert_out  gain=0.5  offset=-5300
  Byte_16 : Outport
  wires:
  BitwiseOR/1 -> Byte_16/1
  UnitConverter/1 -> BitwiseOR/1
  SignalPack/1 -> UnitConverter/1
  UnitConverter1/1 -> SignalPack/1
  convert_out/1 -> UnitConverter1/1
  Fr_EDUAvailBrkRgnTq/1 -> convert_out/1

== system halout/HAL_OUT/CAN1/FD1_VCU3_0x159/Byte_17 ==
  Fr_EDUAvailBrkRgnTq : Inport
  BitwiseOR : simulink/Logic and Bit Operations/Bitwise Operator  logicop=OR  UseBitMask=off  BitMask=bin2dec('11011001')  BitMaskRealWorld=Stored Integer
  SignalPack : FVT_lib/hal/SignalPack  RightShiftCnt=0  BitMask=2^8-1  LeftShiftCnt=0
  UnitConverter : DataTypeConversion  OutDataTypeStr=uint8  RndMeth=Round
  UnitConverter1 : DataTypeConversion  OutDataTypeStr=uint16  RndMeth=Round
  convert_out : FVT_lib/hal/convert_out  gain=0.5  offset=-5300
  Byte_17 : Outport
  wires:
  BitwiseOR/1 -> Byte_17/1
  UnitConverter/1 -> BitwiseOR/1
  SignalPack/1 -> UnitConverter/1
  UnitConverter1/1 -> SignalPack/1
  convert_out/1 -> UnitConverter1/1
  Fr_EDUAvailBrkRgnTq/1 -> convert_out/1

== system halout/HAL_OUT/CAN1/FD1_VCU3_0x159/Byte_18 ==
  Fr_EDURealDrvOrBRgnTq : Inport
  BitwiseOR : simulink/Logic and Bit Operations/Bitwise Operator  logicop=OR  UseBitMask=off  BitMask=bin2dec('11011001')  BitMaskRealWorld=Stored Integer
  SignalPack : FVT_lib/hal/SignalPack  RightShiftCnt=8  BitMask=2^8-1  LeftShiftCnt=0
  UnitConverter : DataTypeConversion  OutDataTypeStr=uint8  RndMeth=Round
  UnitConverter1 : DataTypeConversion  OutDataTypeStr=uint16  RndMeth=Round
  convert_out : FVT_lib/hal/convert_out  gain=0.5  offset=-5300
  Byte_18 : Outport
  wires:
  BitwiseOR/1 -> Byte_18/1
  UnitConverter/1 -> BitwiseOR/1
  SignalPack/1 -> UnitConverter/1
  UnitConverter1/1 -> SignalPack/1
  convert_out/1 -> UnitConverter1/1
  Fr_EDURealDrvOrBRgnTq/1 -> convert_out/1

== system halout/HAL_OUT/CAN1/FD1_VCU3_0x159/Byte_19 ==
  Fr_EDURealDrvOrBRgnTq : Inport
  BitwiseOR : simulink/Logic and Bit Operations/Bitwise Operator  logicop=OR  UseBitMask=off  BitMask=bin2dec('11011001')  BitMaskRealWorld=Stored Integer
  SignalPack : FVT_lib/hal/SignalPack  RightShiftCnt=0  BitMask=2^8-1  LeftShiftCnt=0
  UnitConverter : DataTypeConversion  OutDataTypeStr=uint8  RndMeth=Round
  UnitConverter1 : DataTypeConversion  OutDataTypeStr=uint16  RndMeth=Round
  convert_out : FVT_lib/hal/convert_out  gain=0.5  offset=-5300
  Byte_19 : Outport
  wires:
  BitwiseOR/1 -> Byte_19/1
  UnitConverter/1 -> BitwiseOR/1
  SignalPack/1 -> UnitConverter/1
  UnitConverter1/1 -> SignalPack/1
  convert_out/1 -> UnitConverter1/1
  Fr_EDURealDrvOrBRgnTq/1 -> convert_out/1

== system halout/HAL_OUT/CAN1/FD1_VCU3_0x159/Byte_3 ==
  Fr_EDUSpdValid : Inport
  Fr_RgnDecrSta : Inport  Port=2
  Fr_RgnPermSta : Inport  Port=3
  RgnAbnorSta : Inport  Port=4
  Rr_EDUSpdValid : Inport  Port=5
  Rr_RgnDecrSta : Inport  Port=6
  Rr_RgnPermSta : Inport  Port=7
  BitwiseOR : simulink/Logic and Bit Operations/Bitwise Operator  logicop=OR  UseBitMask=off  NumInputPorts=7  BitMask=bin2dec('11011001')  BitMaskRealWorld=Stored Integer
  SignalPack : FVT_lib/hal/SignalPack  RightShiftCnt=0  BitMask=2^1-1  LeftShiftCnt=6
  SignalPack1 : FVT_lib/hal/SignalPack  RightShiftCnt=0  BitMask=2^1-1  LeftShiftCnt=3
  SignalPack2 : FVT_lib/hal/SignalPack  RightShiftCnt=0  BitMask=2^1-1  LeftShiftCnt=1
  SignalPack3 : FVT_lib/hal/SignalPack  RightShiftCnt=0  BitMask=2^1-1  LeftShiftCnt=4
  SignalPack4 : FVT_lib/hal/SignalPack  RightShiftCnt=0  BitMask=2^1-1  LeftShiftCnt=5
  SignalPack5 : FVT_lib/hal/SignalPack  RightShiftCnt=0  BitMask=2^1-1  LeftShiftCnt=2
  SignalPack6 : FVT_lib/hal/SignalPack  RightShiftCnt=0  BitMask=2^1-1  LeftShiftCnt=0
  UnitConverter{,1..13} (14 alike) : DataTypeConversion  OutDataTypeStr=uint8  RndMeth=Round
  Byte_3 : Outport
  wires:
  BitwiseOR/1 -> Byte_3/1
  UnitConverter/1 -> BitwiseOR/1
  SignalPack/1 -> UnitConverter/1
  UnitConverter1/1 -> SignalPack/1
  Fr_EDUSpdValid/1 -> UnitConverter1/1
  UnitConverter2/1 -> BitwiseOR/2
  SignalPack1/1 -> UnitConverter2/1
  UnitConverter3/1 -> SignalPack1/1
  Fr_RgnDecrSta/1 -> UnitConverter3/1
  UnitConverter4/1 -> BitwiseOR/3
  SignalPack2/1 -> UnitConverter4/1
  UnitConverter5/1 -> SignalPack2/1
  Fr_RgnPermSta/1 -> UnitConverter5/1
  UnitConverter6/1 -> BitwiseOR/4
  SignalPack3/1 -> UnitConverter6/1
  UnitConverter7/1 -> SignalPack3/1
  RgnAbnorSta/1 -> UnitConverter7/1
  UnitConverter8/1 -> BitwiseOR/5
  SignalPack4/1 -> UnitConverter8/1
  UnitConverter9/1 -> SignalPack4/1
  Rr_EDUSpdValid/1 -> UnitConverter9/1
  UnitConverter10/1 -> BitwiseOR/6
  SignalPack5/1 -> UnitConverter10/1
  UnitConverter11/1 -> SignalPack5/1
  Rr_RgnDecrSta/1 -> UnitConverter11/1
  UnitConverter12/1 -> BitwiseOR/7
  SignalPack6/1 -> UnitConverter12/1
  UnitConverter13/1 -> SignalPack6/1
  Rr_RgnPermSta/1 -> UnitConverter13/1

== system halout/HAL_OUT/CAN1/FD1_VCU3_0x159/Byte_4 ==
  EquivAccPedalSWSta : Inport
  PTCS_PermSta : Inport  Port=2
  Rr_EDUSpd : Inport  Port=3
  BitwiseOR : simulink/Logic and Bit Operations/Bitwise Operator  logicop=OR  UseBitMask=off  NumInputPorts=3  BitMask=bin2dec('11011001')  BitMaskRealWorld=Stored Integer
  SignalPack : FVT_lib/hal/SignalPack  RightShiftCnt=0  BitMask=2^1-1  LeftShiftCnt=6
  SignalPack1 : FVT_lib/hal/SignalPack  RightShiftCnt=0  BitMask=2^1-1  LeftShiftCnt=7
  SignalPack2 : FVT_lib/hal/SignalPack  RightShiftCnt=8  BitMask=2^4-1  LeftShiftCnt=0
  UnitConverter{,1..4} (5 alike) : DataTypeConversion  OutDataTypeStr=uint8  RndMeth=Round
  UnitConverter5 : DataTypeConversion  OutDataTypeStr=uint16  RndMeth=Round
  convert_out : FVT_lib/hal/convert_out  gain=1  offset=-2000
  Byte_4 : Outport
  wires:
  BitwiseOR/1 -> Byte_4/1
  UnitConverter/1 -> BitwiseOR/1
  SignalPack/1 -> UnitConverter/1
  UnitConverter1/1 -> SignalPack/1
  EquivAccPedalSWSta/1 -> UnitConverter1/1
  UnitConverter2/1 -> BitwiseOR/2
  SignalPack1/1 -> UnitConverter2/1
  UnitConverter3/1 -> SignalPack1/1
  PTCS_PermSta/1 -> UnitConverter3/1
  UnitConverter4/1 -> BitwiseOR/3
  SignalPack2/1 -> UnitConverter4/1
  UnitConverter5/1 -> SignalPack2/1
  convert_out/1 -> UnitConverter5/1
  Rr_EDUSpd/1 -> convert_out/1

== system halout/HAL_OUT/CAN1/FD1_VCU3_0x159/Byte_5 ==
  Rr_EDUSpd : Inport
  BitwiseOR : simulink/Logic and Bit Operations/Bitwise Operator  logicop=OR  UseBitMask=off  BitMask=bin2dec('11011001')  BitMaskRealWorld=Stored Integer
  SignalPack : FVT_lib/hal/SignalPack  RightShiftCnt=0  BitMask=2^8-1  LeftShiftCnt=0
  UnitConverter : DataTypeConversion  OutDataTypeStr=uint8  RndMeth=Round
  UnitConverter1 : DataTypeConversion  OutDataTypeStr=uint16  RndMeth=Round
  convert_out : FVT_lib/hal/convert_out  gain=1  offset=-2000
  Byte_5 : Outport
  wires:
  BitwiseOR/1 -> Byte_5/1
  UnitConverter/1 -> BitwiseOR/1
  SignalPack/1 -> UnitConverter/1
  UnitConverter1/1 -> SignalPack/1
  convert_out/1 -> UnitConverter1/1
  Rr_EDUSpd/1 -> convert_out/1

== system halout/HAL_OUT/CAN1/FD1_VCU3_0x159/Byte_6 ==
  Rr_EDURealARgnTq : Inport
  BitwiseOR : simulink/Logic and Bit Operations/Bitwise Operator  logicop=OR  UseBitMask=off  BitMask=bin2dec('11011001')  BitMaskRealWorld=Stored Integer
  SignalPack : FVT_lib/hal/SignalPack  RightShiftCnt=8  BitMask=2^8-1  LeftShiftCnt=0
  UnitConverter : DataTypeConversion  OutDataTypeStr=uint8  RndMeth=Round
  UnitConverter1 : DataTypeConversion  OutDataTypeStr=uint16  RndMeth=Round
  convert_out : FVT_lib/hal/convert_out  gain=1  offset=-5300
  Byte_6 : Outport
  wires:
  BitwiseOR/1 -> Byte_6/1
  UnitConverter/1 -> BitwiseOR/1
  SignalPack/1 -> UnitConverter/1
  UnitConverter1/1 -> SignalPack/1
  convert_out/1 -> UnitConverter1/1
  Rr_EDURealARgnTq/1 -> convert_out/1

== system halout/HAL_OUT/CAN1/FD1_VCU3_0x159/Byte_7 ==
  Rr_EDURealARgnTq : Inport
  BitwiseOR : simulink/Logic and Bit Operations/Bitwise Operator  logicop=OR  UseBitMask=off  BitMask=bin2dec('11011001')  BitMaskRealWorld=Stored Integer
  SignalPack : FVT_lib/hal/SignalPack  RightShiftCnt=0  BitMask=2^8-1  LeftShiftCnt=0
  UnitConverter : DataTypeConversion  OutDataTypeStr=uint8  RndMeth=Round
  UnitConverter1 : DataTypeConversion  OutDataTypeStr=uint16  RndMeth=Round
  convert_out : FVT_lib/hal/convert_out  gain=1  offset=-5300
  Byte_7 : Outport
  wires:
  BitwiseOR/1 -> Byte_7/1
  UnitConverter/1 -> BitwiseOR/1
  SignalPack/1 -> UnitConverter/1
  UnitConverter1/1 -> SignalPack/1
  convert_out/1 -> UnitConverter1/1
  Rr_EDURealARgnTq/1 -> convert_out/1

== system halout/HAL_OUT/CAN1/FD1_VCU3_0x159/Byte_8 ==
  Rr_EDUAvailBrkRgnTq : Inport
  BitwiseOR : simulink/Logic and Bit Operations/Bitwise Operator  logicop=OR  UseBitMask=off  BitMask=bin2dec('11011001')  BitMaskRealWorld=Stored Integer
  SignalPack : FVT_lib/hal/SignalPack  RightShiftCnt=8  BitMask=2^8-1  LeftShiftCnt=0
  UnitConverter : DataTypeConversion  OutDataTypeStr=uint8  RndMeth=Round
  UnitConverter1 : DataTypeConversion  OutDataTypeStr=uint16  RndMeth=Round
  convert_out : FVT_lib/hal/convert_out  gain=0.5  offset=-5300
  Byte_8 : Outport
  wires:
  BitwiseOR/1 -> Byte_8/1
  UnitConverter/1 -> BitwiseOR/1
  SignalPack/1 -> UnitConverter/1
  UnitConverter1/1 -> SignalPack/1
  convert_out/1 -> UnitConverter1/1
  Rr_EDUAvailBrkRgnTq/1 -> convert_out/1

== system halout/HAL_OUT/CAN1/FD1_VCU3_0x159/Byte_9 ==
  Rr_EDUAvailBrkRgnTq : Inport
  BitwiseOR : simulink/Logic and Bit Operations/Bitwise Operator  logicop=OR  UseBitMask=off  BitMask=bin2dec('11011001')  BitMaskRealWorld=Stored Integer
  SignalPack : FVT_lib/hal/SignalPack  RightShiftCnt=0  BitMask=2^8-1  LeftShiftCnt=0
  UnitConverter : DataTypeConversion  OutDataTypeStr=uint8  RndMeth=Round
  UnitConverter1 : DataTypeConversion  OutDataTypeStr=uint16  RndMeth=Round
  convert_out : FVT_lib/hal/convert_out  gain=0.5  offset=-5300
  Byte_9 : Outport
  wires:
  BitwiseOR/1 -> Byte_9/1
  UnitConverter/1 -> BitwiseOR/1
  SignalPack/1 -> UnitConverter/1
  UnitConverter1/1 -> SignalPack/1
  convert_out/1 -> UnitConverter1/1
  Rr_EDUAvailBrkRgnTq/1 -> convert_out/1

== system halout/HAL_OUT/CAN1/FD1_VCU3_0x159/CRC8_IfAction_Tx ==
  CAN_E2E_flg : Inport
  DataID1 : Inport  Port=2
  DataID2 : Inport  Port=3
  RawData : Inport  Port=4
  Data Type Conversion : DataTypeConversion  OutDataTypeStr=uint8
  If : If
  If Action Subsystem : Subsystem  TreatAsAtomicUnit=on
  If Action Subsystem1 : Subsystem  TreatAsAtomicUnit=on
  Merge : Merge
  CRC8 : Outport
  wires:
  If/2 -> If Action Subsystem/Action
  If/1 -> If Action Subsystem1/Action
  CAN_E2E_flg/1 -> [CAN_E2E_flg]
  DataID1/1 -> [DataID1]
  DataID2/1 -> [DataID2]
  RawData/1 -> [RawData]
  [CAN_E2E_flg] -> Data Type Conversion/1
  [DataID1] -> If Action Subsystem1/1(CAN_E2E_ID1)
  [DataID2] -> If Action Subsystem1/2(CAN_E2E_ID2)
  [RawData] -> If Action Subsystem1/3(Byte1)
  [RawData] -> If Action Subsystem/1(Byte1)
  If Action Subsystem1/1(CRC8_E2EResult) -> Merge/1
  If Action Subsystem/1(CRC8_Result) -> Merge/2
  Merge/1 -> CRC8/1
  Data Type Conversion/1 -> If/1

== system halout/HAL_OUT/CAN1/FD1_VCU3_0x159/CSVCU3CAN1 ==
  CSVCU3CAN1 : Inport
  Data Type Conversion : DataTypeConversion  OutDataTypeStr=uint8  RndMeth=Round
  CAN1_CS_VCU3_CAN1 : Outport
  wires:
  Data Type Conversion/1 -> CAN1_CS_VCU3_CAN1/1
  CSVCU3CAN1/1 -> Data Type Conversion/1

== system halout/HAL_OUT/CAN1/FD1_VCU3_0x159/EquivAccPedalSWSta ==
  EquivAccPedalSWSta : Inport
  Data Type Conversion : DataTypeConversion  OutDataTypeStr=uint8  RndMeth=Round
  CAN1_EquivAccPedalSWSta : Outport
  wires:
  Data Type Conversion/1 -> CAN1_EquivAccPedalSWSta/1
  EquivAccPedalSWSta/1 -> Data Type Conversion/1

== system halout/HAL_OUT/CAN1/FD1_VCU3_0x159/FrEDUAvailBrkRgnTq ==
  FrEDUAvailBrkRgnTq : Inport
  Data Type Conversion : DataTypeConversion  OutDataTypeStr=uint16  RndMeth=Round
  convert_out : FVT_lib/hal/convert_out  gain=0.5  offset=-5300
  CAN1_Fr_EDUAvailBrkRgnTq : Outport
  wires:
  Data Type Conversion/1 -> CAN1_Fr_EDUAvailBrkRgnTq/1
  convert_out/1 -> Data Type Conversion/1
  FrEDUAvailBrkRgnTq/1 -> convert_out/1

== system halout/HAL_OUT/CAN1/FD1_VCU3_0x159/FrEDUAvailBrkRgnTqValid ==
  FrEDUAvailBrkRgnTqValid : Inport
  Data Type Conversion : DataTypeConversion  OutDataTypeStr=uint8  RndMeth=Round
  CAN1_Fr_EDUAvailBrkRgnTqValid : Outport
  wires:
  Data Type Conversion/1 -> CAN1_Fr_EDUAvailBrkRgnTqValid/1
  FrEDUAvailBrkRgnTqValid/1 -> Data Type Conversion/1

== system halout/HAL_OUT/CAN1/FD1_VCU3_0x159/FrEDURealARgnTq ==
  FrEDURealARgnTq : Inport
  Data Type Conversion : DataTypeConversion  OutDataTypeStr=uint16  RndMeth=Round
  convert_out : FVT_lib/hal/convert_out  gain=1  offset=-5300
  CAN1_Fr_EDURealARgnTq : Outport
  wires:
  Data Type Conversion/1 -> CAN1_Fr_EDURealARgnTq/1
  convert_out/1 -> Data Type Conversion/1
  FrEDURealARgnTq/1 -> convert_out/1

== system halout/HAL_OUT/CAN1/FD1_VCU3_0x159/FrEDURealDrvOrBRgnTq ==
  FrEDURealDrvOrBRgnTq : Inport
  Data Type Conversion : DataTypeConversion  OutDataTypeStr=uint16  RndMeth=Round
  convert_out : FVT_lib/hal/convert_out  gain=0.5  offset=-5300
  CAN1_Fr_EDURealDrvOrBRgnTq : Outport
  wires:
  Data Type Conversion/1 -> CAN1_Fr_EDURealDrvOrBRgnTq/1
  convert_out/1 -> Data Type Conversion/1
  FrEDURealDrvOrBRgnTq/1 -> convert_out/1

== system halout/HAL_OUT/CAN1/FD1_VCU3_0x159/FrEDUSpd ==
  FrEDUSpd : Inport
  Data Type Conversion : DataTypeConversion  OutDataTypeStr=uint16  RndMeth=Round
  convert_out : FVT_lib/hal/convert_out  gain=1  offset=-2000
  CAN1_Fr_EDUSpd : Outport
  wires:
  Data Type Conversion/1 -> CAN1_Fr_EDUSpd/1
  convert_out/1 -> Data Type Conversion/1
  FrEDUSpd/1 -> convert_out/1

== system halout/HAL_OUT/CAN1/FD1_VCU3_0x159/FrEDUSpdValid ==
  FrEDUSpdValid : Inport
  Data Type Conversion : DataTypeConversion  OutDataTypeStr=uint8  RndMeth=Round
  CAN1_Fr_EDUSpdValid : Outport
  wires:
  Data Type Conversion/1 -> CAN1_Fr_EDUSpdValid/1
  FrEDUSpdValid/1 -> Data Type Conversion/1

== system halout/HAL_OUT/CAN1/FD1_VCU3_0x159/FrRgnDecrSta ==
  FrRgnDecrSta : Inport
  Data Type Conversion : DataTypeConversion  OutDataTypeStr=uint8  RndMeth=Round
  CAN1_Fr_RgnDecrSta : Outport
  wires:
  Data Type Conversion/1 -> CAN1_Fr_RgnDecrSta/1
  FrRgnDecrSta/1 -> Data Type Conversion/1

== system halout/HAL_OUT/CAN1/FD1_VCU3_0x159/FrRgnPermSta ==
  FrRgnPermSta : Inport
  Data Type Conversion : DataTypeConversion  OutDataTypeStr=uint8  RndMeth=Round
  CAN1_Fr_RgnPermSta : Outport
  wires:
  Data Type Conversion/1 -> CAN1_Fr_RgnPermSta/1
  FrRgnPermSta/1 -> Data Type Conversion/1

== system halout/HAL_OUT/CAN1/FD1_VCU3_0x159/PTCSPermSta ==
  PTCSPermSta : Inport
  Data Type Conversion : DataTypeConversion  OutDataTypeStr=uint8  RndMeth=Round
  CAN1_PTCS_PermSta : Outport
  wires:
  Data Type Conversion/1 -> CAN1_PTCS_PermSta/1
  PTCSPermSta/1 -> Data Type Conversion/1

== system halout/HAL_OUT/CAN1/FD1_VCU3_0x159/RCVCU3CAN1 ==
  RCVCU3CAN1 : Inport
  Data Type Conversion : DataTypeConversion  OutDataTypeStr=uint8  RndMeth=Round
  CAN1_RC_VCU3_CAN1 : Outport
  wires:
  Data Type Conversion/1 -> CAN1_RC_VCU3_CAN1/1
  RCVCU3CAN1/1 -> Data Type Conversion/1

== system halout/HAL_OUT/CAN1/FD1_VCU3_0x159/RgnAbnorSta ==
  RgnAbnorSta : Inport
  Data Type Conversion : DataTypeConversion  OutDataTypeStr=uint8  RndMeth=Round
  CAN1_RgnAbnorSta : Outport
  wires:
  Data Type Conversion/1 -> CAN1_RgnAbnorSta/1
  RgnAbnorSta/1 -> Data Type Conversion/1

== system halout/HAL_OUT/CAN1/FD1_VCU3_0x159/RrEDUAvailBrkRgnTq ==
  RrEDUAvailBrkRgnTq : Inport
  Data Type Conversion : DataTypeConversion  OutDataTypeStr=uint16  RndMeth=Round
  convert_out : FVT_lib/hal/convert_out  gain=0.5  offset=-5300
  CAN1_Rr_EDUAvailBrkRgnTq : Outport
  wires:
  Data Type Conversion/1 -> CAN1_Rr_EDUAvailBrkRgnTq/1
  convert_out/1 -> Data Type Conversion/1
  RrEDUAvailBrkRgnTq/1 -> convert_out/1

== system halout/HAL_OUT/CAN1/FD1_VCU3_0x159/RrEDUAvailBrkRgnTqValid ==
  RrEDUAvailBrkRgnTqValid : Inport
  Data Type Conversion : DataTypeConversion  OutDataTypeStr=uint8  RndMeth=Round
  CAN1_Rr_EDUAvailBrkRgnTqValid : Outport
  wires:
  Data Type Conversion/1 -> CAN1_Rr_EDUAvailBrkRgnTqValid/1
  RrEDUAvailBrkRgnTqValid/1 -> Data Type Conversion/1

== system halout/HAL_OUT/CAN1/FD1_VCU3_0x159/RrEDURealARgnTq ==
  RrEDURealARgnTq : Inport
  Data Type Conversion : DataTypeConversion  OutDataTypeStr=uint16  RndMeth=Round
  convert_out : FVT_lib/hal/convert_out  gain=1  offset=-5300
  CAN1_Rr_EDURealARgnTq : Outport
  wires:
  Data Type Conversion/1 -> CAN1_Rr_EDURealARgnTq/1
  convert_out/1 -> Data Type Conversion/1
  RrEDURealARgnTq/1 -> convert_out/1
